simulink model "Week1_Q3"  (R2020b)
settings: Solver=VariableStepAuto  StartTime=0.0  StopTime=10.0  RelTol=1e-3
settings Model: Creator=DELL  LastModifiedBy=DELL

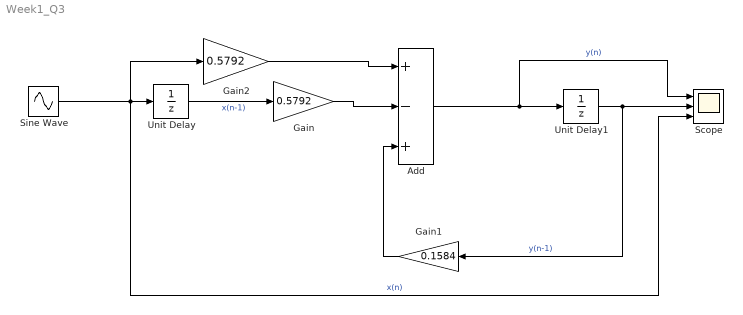
== system Week1_Q3 ==
  Add : Sum  Inputs=+-+
  Gain : Gain  Gain=0.5792
  Gain1 : Gain  Gain=0.1584
  Gain2 : Gain  Gain=0.5792
  Scope : Scope  NumInputPorts=3
  Sine Wave : Sin  Frequency=2*pi*800  SampleTime=1/5000
  Unit Delay : UnitDelay  SampleTime=-1  HasFrameUpgradeWarning=on
  Unit Delay1 : UnitDelay  SampleTime=-1  HasFrameUpgradeWarning=on
  wires:
  Sine Wave/1 -> Scope/3, Unit Delay/1, Gain2/1  "x(n)"
  Gain2/1 -> Add/1
  Unit Delay/1 -> Gain/1  "x(n-1)"
  Gain/1 -> Add/2
  Add/1 -> Scope/1, Unit Delay1/1  "y(n)"
  Unit Delay1/1 -> Gain1/1, Scope/2  "y(n-1)"
  Gain1/1 -> Add/3
